simulink model "MojModel"  (R2021b)
settings: Solver=VariableStepAuto  StartTime=0.0  StopTime=10.0  RelTol=1e-3
undefined symbols (not defined in the file): A, x0
settings Model: Creator=student  LastModifiedBy=szczy

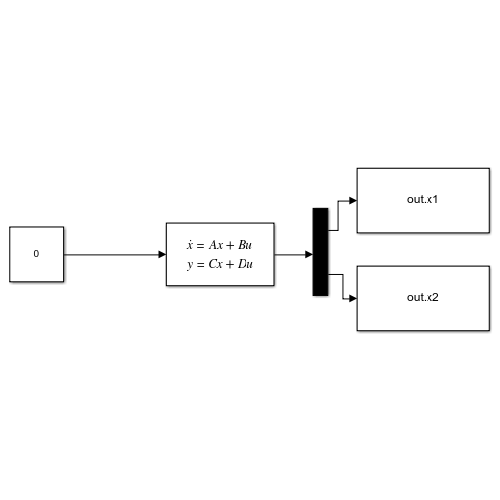
[thumbnail: Simulink's stored preview of the top-level diagram]
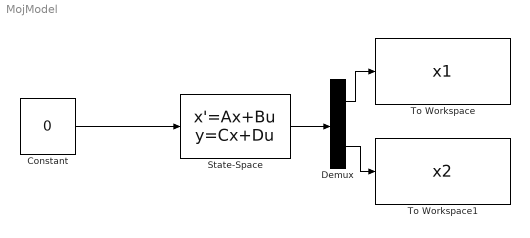
== system MojModel ==
  Constant : Constant  Value=0
  Demux : Demux  Outputs=2
  State-Space : StateSpace  A=A  B=[0; 0]  C=[1 0; 0 1]  D=[0; 0]  InitialCondition=x0
  To Workspace : ToWorkspace  VariableName=x1  SampleTime=-1
  To Workspace1 : ToWorkspace  VariableName=x2  SampleTime=-1
  wires:
  Constant/1 -> State-Space/1
  Demux/1 -> To Workspace/1
  Demux/2 -> To Workspace1/1
  State-Space/1 -> Demux/1
